simulink model "mp1"  (R2018b)
settings: Solver=VariableStepAuto  StartTime=0.0  StopTime=10.0  RelTol=1e-3
values from neighbouring files (symbols this model uses):
  b = 54.2e-6    (= 5.42e-05)    [Untitled_M65.m]
  d = 1.1e-6    (= 1.1e-06)    [Untitled_M65.m]
  g = 9.81    [Untitled_M65.m]
  I = 1.08e-6    (= 1.08e-06)    [Untitled_M65.m]
  Ix = 0.008    [Untitled_M65.m]
  Iy = 0.008    [Untitled_M65.m]
  Iz = 0.142    [Untitled_M65.m]
  L = 0.24    [Untitled_M65.m]
  m = 1    [Untitled_M65.m]
  Pos_z0 = 150    [Untitled_M65.m]
libraries: mpclib x2
settings Model: Creator=z2822  LastModifiedBy=z2822

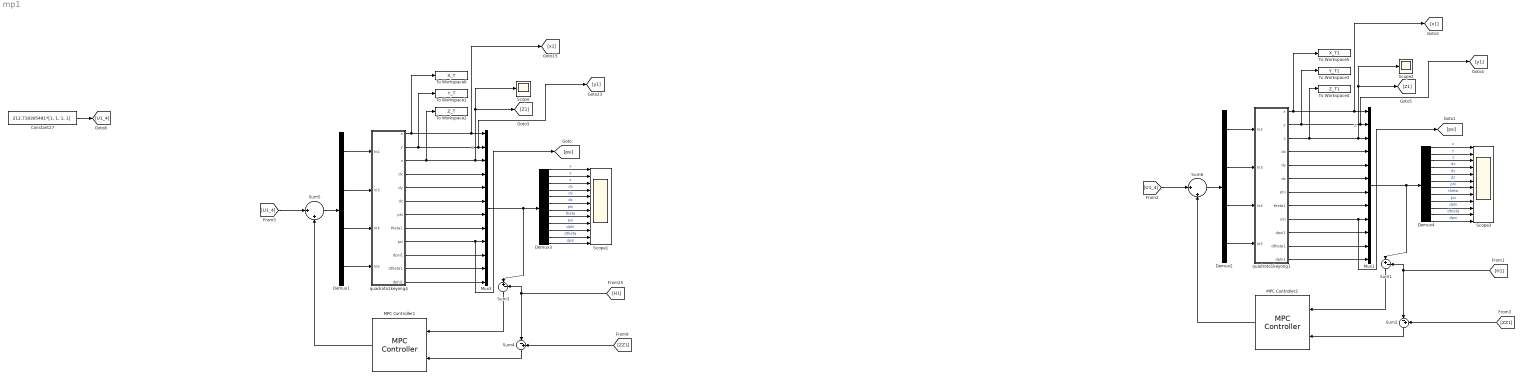
== system mp1 ==
  Constant27 : Constant  Value=212.718305491*[1, 1, 1, 1]
  Demux1 : Demux
  Demux2 : Demux
  Demux3 : Demux  Outputs=12
  Demux4 : Demux  Outputs=12
  MPC Controller1 : mpclib/MPC Controller  SCDEnableBlockLinearizationSpecification=on  mpcobj=mpc1  is_multiple=0  enable_value=0  return_u0=off  updateMPCinCallerWorkspace=on  md_inport=off  mv_inport=off  return_cost=off  return_mvseq=off  return_qpstatus=off  return_xseq=off  return_state=off  return_ovseq=off  state_inport=off  umin_inport=off  umax_inport=off  ymin_inport=off  ymax_inport=off  cc_inport=off  ywt_inport=off  uwt_inport=off  duwt_inport=off  rhoeps_inport=off  uref_inport=off  n_ts=0.83  n_p=23  n_mv=4  n_md=0  n_ud=0  n_mo=12  n_uo=0  BlockDataType=double  SampleTimeInherited=off  switch_inport=off
  MPC Controller2 : mpclib/MPC Controller  SCDEnableBlockLinearizationSpecification=on  mpcobj=mpc1  is_multiple=0  enable_value=0  return_u0=off  updateMPCinCallerWorkspace=on  md_inport=off  mv_inport=off  return_cost=off  return_mvseq=off  return_qpstatus=off  return_xseq=off  return_state=off  return_ovseq=off  state_inport=off  umin_inport=off  umax_inport=off  ymin_inport=off  ymax_inport=off  cc_inport=off  ywt_inport=off  uwt_inport=off  duwt_inport=off  rhoeps_inport=off  uref_inport=off  n_ts=0.83  n_p=23  n_mv=4  n_md=0  n_ud=0  n_mo=12  n_uo=0  BlockDataType=double  SampleTimeInherited=off  switch_inport=off
  Mux1 : Mux  Inputs=12
  Mux3 : Mux  Inputs=12
  Scope : Scope
  Scope1 : Scope  NumInputPorts=12
  Scope2 : Scope
  Scope3 : Scope  NumInputPorts=12
  Sum1 : Sum  Inputs=|+-
  Sum2 : Sum  Inputs=|-+
  Sum3 : Sum  Inputs=|+-
  Sum4 : Sum  Inputs=|-+
  Sum5 : Sum  Inputs=||+|+
  Sum6 : Sum  Inputs=||+|+
  To Workspace1 : ToWorkspace  VariableName=Y_T  SaveFormat=Timeseries  SampleTime=-1
  To Workspace2 : ToWorkspace  VariableName=Z_T  SaveFormat=Timeseries  SampleTime=-1
  To Workspace3 : ToWorkspace  VariableName=Y_T1  SaveFormat=Timeseries  SampleTime=-1
  To Workspace4 : ToWorkspace  VariableName=Z_T1  SaveFormat=Timeseries  SampleTime=-1
  To Workspace5 : ToWorkspace  VariableName=X_T1  SaveFormat=Timeseries  SampleTime=-1
  To Workspace6 : ToWorkspace  VariableName=X_T  SaveFormat=Timeseries  SampleTime=-1
  quadroto1keyong1 : Subsystem
  quadroto1keyong4 : Subsystem
  wires:
  Demux3/8 -> Scope1/8  "theta"
  Demux3/6 -> Scope1/6  "dz"
  Demux3/12 -> Scope1/12  "dpsi"
  quadroto1keyong4/12(dphi1) -> Mux3/12
  Demux3/4 -> Scope1/4  "dx"
  Demux3/9 -> Scope1/9  "psi"
  Demux3/10 -> Scope1/10  "dphi"
  Demux3/11 -> Scope1/11  "dtheta"
  quadroto1keyong4/5(dy) -> Mux3/5
  quadroto1keyong4/11(dtheta1) -> Mux3/11
  quadroto1keyong4/10(dpsi1) -> Mux3/10
  MPC Controller1/1 -> Sum5/2
  Demux3/5 -> Scope1/5  "dy"
  quadroto1keyong4/9(psi) -> [psi], Mux3/9
  Demux1/1 -> quadroto1keyong4/1(In2)
  quadroto1keyong4/2(y) -> To Workspace1/1, Mux3/2, [y1]
  [ZZ1] -> Sum4/2
  Sum4/1 -> MPC Controller1/2
  Demux1/4 -> quadroto1keyong4/4(In5)
  Demux3/1 -> Scope1/1  "x"
  Demux3/3 -> Scope1/3  "z"
  [H1] -> Sum4/1, Sum3/2
  quadroto1keyong4/7(phi) -> Mux3/7
  quadroto1keyong4/4(dx) -> Mux3/4
  Demux1/3 -> quadroto1keyong4/3(In4)
  Sum5/1 -> Demux1/1
  quadroto1keyong4/6(dz) -> Mux3/6
  quadroto1keyong4/8(theta1) -> Mux3/8
  Sum3/1 -> MPC Controller1/1
  Mux3/1 -> Sum3/1, Demux3/1
  Demux3/2 -> Scope1/2  "y"
  quadroto1keyong4/3(z) -> To Workspace2/1, Mux3/3, Scope/1, [Z1]  "Z"
  [U1_4] -> Sum5/1
  Demux3/7 -> Scope1/7  "phi"
  quadroto1keyong4/1(x) -> To Workspace6/1, Mux3/1, [x1]
  Demux1/2 -> quadroto1keyong4/2(In3)
  quadroto1keyong1/1(x) -> To Workspace5/1, Mux1/1, [x1]
  Demux4/7 -> Scope3/7  "phi"
  quadroto1keyong1/8(theta1) -> Mux1/8
  quadroto1keyong1/6(dz) -> Mux1/6
  Sum6/1 -> Demux2/1
  Demux2/3 -> quadroto1keyong1/3(In4)
  [U1_4] -> Sum6/1
  Sum1/1 -> MPC Controller2/1
  Demux4/1 -> Scope3/1  "x"
  quadroto1keyong1/3(z) -> To Workspace4/1, Mux1/3, Scope2/1, [Z1]  "Z"
  Demux4/3 -> Scope3/3  "z"
  quadroto1keyong1/4(dx) -> Mux1/4
  [ZZ1] -> Sum2/2
  Mux1/1 -> Sum1/1, Demux4/1
  quadroto1keyong1/7(phi) -> Mux1/7
  quadroto1keyong1/2(y) -> To Workspace3/1, Mux1/2, [y1]
  Demux4/9 -> Scope3/9  "psi"
  quadroto1keyong1/5(dy) -> Mux1/5
  Demux4/2 -> Scope3/2  "y"
  quadroto1keyong1/11(dtheta1) -> Mux1/11
  Demux2/1 -> quadroto1keyong1/1(In2)
  Demux4/5 -> Scope3/5  "dy"
  [H1] -> Sum2/1, Sum1/2
  Demux2/4 -> quadroto1keyong1/4(In5)
  MPC Controller2/1 -> Sum6/2
  Demux2/2 -> quadroto1keyong1/2(In3)
  quadroto1keyong1/10(dpsi1) -> Mux1/10
  Demux4/10 -> Scope3/10  "dphi"
  Demux4/11 -> Scope3/11  "dtheta"
  Demux4/6 -> Scope3/6  "dz"
  Sum2/1 -> MPC Controller2/2
  quadroto1keyong1/12(dphi1) -> Mux1/12
  quadroto1keyong1/9(psi) -> [psi], Mux1/9
  Demux4/12 -> Scope3/12  "dpsi"
  Demux4/4 -> Scope3/4  "dx"
  Demux4/8 -> Scope3/8  "theta"
  Constant27/1 -> [U1_4]

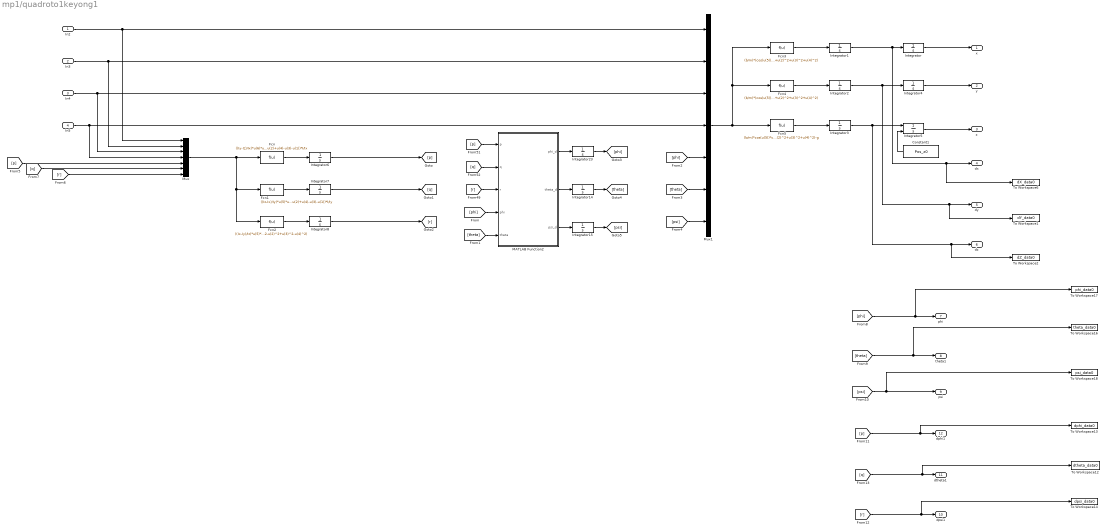
== system mp1/quadroto1keyong1 ==
  In2 : Inport
  In3 : Inport  Port=2
  In4 : Inport  Port=3
  In5 : Inport  Port=4
  Constant1 : Constant  Value=Pos_z0
  Fcn : Fcn  Expr=((Iy-Iz)/Ix)*u(6)*u(7)+(b*L/Ix)*(u(4)^2-u(2)^2)-u(6)*(u(2)+u(4)-u(3)-u(1))*I/Ix
  Fcn1 : Fcn  Expr=((Iz-Ix)/Iy)*u(5)*u(7)+(b*L/Iy)*(u(3)^2-u(1)^2)-u(5)*(u(2)+u(4)-u(3)-u(1))*I/Iy
  Fcn2 : Fcn  Expr=((Ix-Iy)/Iz)*u(5)*u(6)+(d/Iz)*(u(1)^2-u(2)^2+u(3)^2-u(4)^2)
  Fcn3 : Fcn  Expr=(b/m)*(cos(u(5))*sin(u(6))*cos(u(7))+sin(u(5))*sin(u(7)))*(u(1)^2+u(2)^2+u(3)^2+u(4)^2)
  Fcn4 : Fcn  Expr=(b/m)*(cos(u(5))*sin(u(6))*sin(u(7))-sin(u(5))*cos(u(7)))*(u(1)^2+u(2)^2+u(3)^2+u(4)^2)
  Fcn5 : Fcn  Expr=(b/m)*cos(u(5))*cos(u(6))*(u(1)^2+u(2)^2+u(3)^2+u(4)^2)-g
  Integrator{,1..4,6..8,14..15,23} (11 alike) : Integrator
  Integrator5 : Integrator  InitialConditionSource=external
  MATLAB Function2 : MATLAB Function  TreatAsAtomicUnit=on
  Mux : Mux  Inputs=7
  Mux1 : Mux  Inputs=7
  To Workspace1 : ToWorkspace  VariableName=dY_data0  SaveFormat=Timeseries  SampleTime=-1
  To Workspace12 : ToWorkspace  VariableName=dtheta_data0  SaveFormat=Timeseries  SampleTime=-1
  To Workspace13 : ToWorkspace  VariableName=dphi_data0  SaveFormat=Timeseries  SampleTime=-1
  To Workspace14 : ToWorkspace  VariableName=dpsi_data0  SaveFormat=Timeseries  SampleTime=-1
  To Workspace16 : ToWorkspace  VariableName=theta_data0  SaveFormat=Timeseries  SampleTime=-1
  To Workspace17 : ToWorkspace  VariableName=phi_data0  SaveFormat=Timeseries  SampleTime=-1
  To Workspace18 : ToWorkspace  VariableName=psi_data0  SaveFormat=Timeseries  SampleTime=-1
  To Workspace2 : ToWorkspace  VariableName=dZ_data0  SaveFormat=Timeseries  SampleTime=-1
  To Workspace6 : ToWorkspace  VariableName=dX_data0  SaveFormat=Timeseries  SampleTime=-1
  x : Outport
  y : Outport  Port=2
  z : Outport  Port=3
  dx : Outport  Port=4
  dy : Outport  Port=5
  dz : Outport  Port=6
  phi : Outport  Port=7
  theta1 : Outport  Port=8
  psi : Outport  Port=9
  dpsi1 : Outport  Port=10
  dtheta1 : Outport  Port=11
  dphi1 : Outport  Port=12
  wires:
  Integrator3/1 -> Integrator5/1, dz/1, To Workspace2/1
  Fcn4/1 -> Integrator2/1
  Integrator4/1 -> y/1
  In4/1 -> Mux1/3, Mux/3
  Integrator1/1 -> Integrator/1, To Workspace6/1, dx/1
  Mux/1 -> Fcn/1, Fcn1/1, Fcn2/1
  In3/1 -> Mux1/2, Mux/2
  Integrator5/1 -> z/1
  Mux1/1 -> Fcn3/1, Fcn4/1, Fcn5/1
  Fcn5/1 -> Integrator3/1
  Integrator2/1 -> Integrator4/1, To Workspace1/1, dy/1
  Fcn2/1 -> Integrator8/1
  In5/1 -> Mux/4, Mux1/4
  Fcn/1 -> Integrator6/1
  In2/1 -> Mux/1, Mux1/1
  Fcn1/1 -> Integrator7/1
  Integrator/1 -> x/1
  Fcn3/1 -> Integrator1/1
  Constant1/1 -> Integrator5/2
  [p] -> MATLAB Function2/1(p)
  [phi] -> Mux1/5
  Integrator23/1 -> [phi]
  [theta] -> MATLAB Function2/5(theta)
  [theta] -> Mux1/6
  MATLAB Function2/3(psi_d) -> Integrator15/1
  Integrator15/1 -> [psi]
  MATLAB Function2/2(theta_d) -> Integrator14/1
  [r] -> MATLAB Function2/3(r)
  [psi] -> Mux1/7
  [phi] -> MATLAB Function2/4(phi)
  [q] -> MATLAB Function2/2(q)
  MATLAB Function2/1(phi_d) -> Integrator23/1
  Integrator14/1 -> [theta]
  Integrator6/1 -> [p]
  Integrator7/1 -> [q]
  Integrator8/1 -> [r]
  [psi] -> psi/1, To Workspace18/1
  [phi] -> phi/1, To Workspace17/1
  [q] -> To Workspace12/1, dtheta1/1
  [r] -> To Workspace14/1, dpsi1/1
  [p] -> To Workspace13/1, dphi1/1
  [theta] -> theta1/1, To Workspace16/1
  [r] -> Mux/7
  [p] -> Mux/5
  [q] -> Mux/6

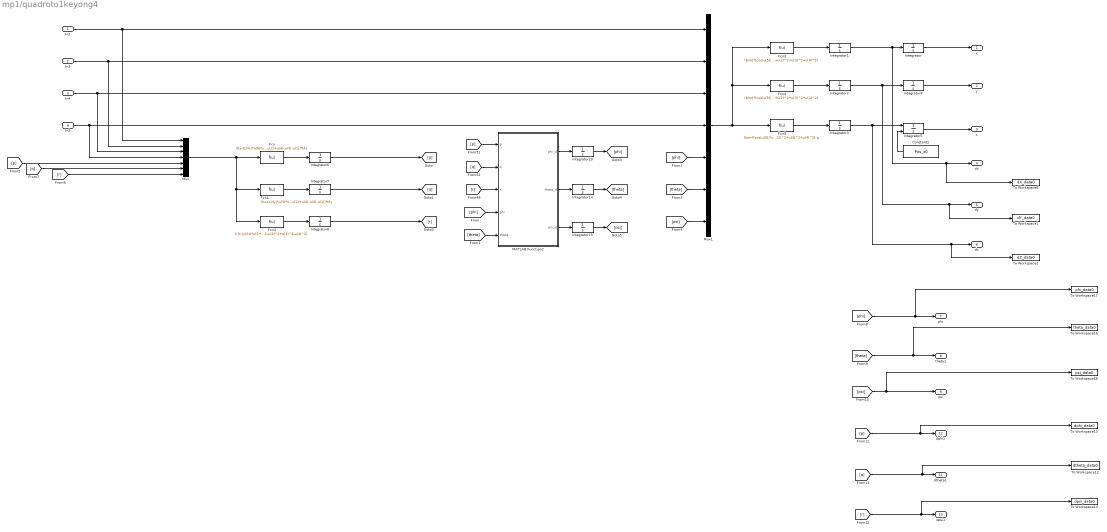
== system mp1/quadroto1keyong4 ==
  In2 : Inport
  In3 : Inport  Port=2
  In4 : Inport  Port=3
  In5 : Inport  Port=4
  Constant1 : Constant  Value=Pos_z0
  Fcn : Fcn  Expr=((Iy-Iz)/Ix)*u(6)*u(7)+(b*L/Ix)*(u(4)^2-u(2)^2)-u(6)*(u(2)+u(4)-u(3)-u(1))*I/Ix
  Fcn1 : Fcn  Expr=((Iz-Ix)/Iy)*u(5)*u(7)+(b*L/Iy)*(u(3)^2-u(1)^2)-u(5)*(u(2)+u(4)-u(3)-u(1))*I/Iy
  Fcn2 : Fcn  Expr=((Ix-Iy)/Iz)*u(5)*u(6)+(d/Iz)*(u(1)^2-u(2)^2+u(3)^2-u(4)^2)
  Fcn3 : Fcn  Expr=(b/m)*(cos(u(5))*sin(u(6))*cos(u(7))+sin(u(5))*sin(u(7)))*(u(1)^2+u(2)^2+u(3)^2+u(4)^2)
  Fcn4 : Fcn  Expr=(b/m)*(cos(u(5))*sin(u(6))*sin(u(7))-sin(u(5))*cos(u(7)))*(u(1)^2+u(2)^2+u(3)^2+u(4)^2)
  Fcn5 : Fcn  Expr=(b/m)*cos(u(5))*cos(u(6))*(u(1)^2+u(2)^2+u(3)^2+u(4)^2)-g
  Integrator{,1..4,6..8,14..15,23} (11 alike) : Integrator
  Integrator5 : Integrator  InitialConditionSource=external
  MATLAB Function2 : MATLAB Function  TreatAsAtomicUnit=on
  Mux : Mux  Inputs=7
  Mux1 : Mux  Inputs=7
  To Workspace1 : ToWorkspace  VariableName=dY_data0  SaveFormat=Timeseries  SampleTime=-1
  To Workspace12 : ToWorkspace  VariableName=dtheta_data0  SaveFormat=Timeseries  SampleTime=-1
  To Workspace13 : ToWorkspace  VariableName=dphi_data0  SaveFormat=Timeseries  SampleTime=-1
  To Workspace14 : ToWorkspace  VariableName=dpsi_data0  SaveFormat=Timeseries  SampleTime=-1
  To Workspace16 : ToWorkspace  VariableName=theta_data0  SaveFormat=Timeseries  SampleTime=-1
  To Workspace17 : ToWorkspace  VariableName=phi_data0  SaveFormat=Timeseries  SampleTime=-1
  To Workspace18 : ToWorkspace  VariableName=psi_data0  SaveFormat=Timeseries  SampleTime=-1
  To Workspace2 : ToWorkspace  VariableName=dZ_data0  SaveFormat=Timeseries  SampleTime=-1
  To Workspace6 : ToWorkspace  VariableName=dX_data0  SaveFormat=Timeseries  SampleTime=-1
  x : Outport
  y : Outport  Port=2
  z : Outport  Port=3
  dx : Outport  Port=4
  dy : Outport  Port=5
  dz : Outport  Port=6
  phi : Outport  Port=7
  theta1 : Outport  Port=8
  psi : Outport  Port=9
  dpsi1 : Outport  Port=10
  dtheta1 : Outport  Port=11
  dphi1 : Outport  Port=12
  wires:
  Integrator3/1 -> Integrator5/1, dz/1, To Workspace2/1
  Fcn4/1 -> Integrator2/1
  Integrator4/1 -> y/1
  In4/1 -> Mux1/3, Mux/3
  Integrator1/1 -> Integrator/1, To Workspace6/1, dx/1
  Mux/1 -> Fcn/1, Fcn1/1, Fcn2/1
  In3/1 -> Mux1/2, Mux/2
  Integrator5/1 -> z/1
  Mux1/1 -> Fcn3/1, Fcn4/1, Fcn5/1
  Fcn5/1 -> Integrator3/1
  Integrator2/1 -> Integrator4/1, To Workspace1/1, dy/1
  Fcn2/1 -> Integrator8/1
  In5/1 -> Mux/4, Mux1/4
  Fcn/1 -> Integrator6/1
  In2/1 -> Mux/1, Mux1/1
  Fcn1/1 -> Integrator7/1
  Integrator/1 -> x/1
  Fcn3/1 -> Integrator1/1
  Constant1/1 -> Integrator5/2
  [p] -> MATLAB Function2/1(p)
  [phi] -> Mux1/5
  Integrator23/1 -> [phi]
  [theta] -> MATLAB Function2/5(theta)
  [theta] -> Mux1/6
  MATLAB Function2/3(psi_d) -> Integrator15/1
  Integrator15/1 -> [psi]
  MATLAB Function2/2(theta_d) -> Integrator14/1
  [r] -> MATLAB Function2/3(r)
  [psi] -> Mux1/7
  [phi] -> MATLAB Function2/4(phi)
  [q] -> MATLAB Function2/2(q)
  MATLAB Function2/1(phi_d) -> Integrator23/1
  Integrator14/1 -> [theta]
  Integrator6/1 -> [p]
  Integrator7/1 -> [q]
  Integrator8/1 -> [r]
  [psi] -> psi/1, To Workspace18/1
  [phi] -> phi/1, To Workspace17/1
  [q] -> To Workspace12/1, dtheta1/1
  [r] -> To Workspace14/1, dpsi1/1
  [p] -> To Workspace13/1, dphi1/1
  [theta] -> theta1/1, To Workspace16/1
  [r] -> Mux/7
  [p] -> Mux/5
  [q] -> Mux/6

== matlab function mp1/quadroto1keyong1/MATLAB Function2 ==
  data: p input; phi_d output; q input; r input; phi input; theta input; theta_d output; psi_d output
function [phi_d, theta_d, psi_d] = fcn(p, q, r, phi, theta)


phi_d = p + q * tan(theta) * sin(phi) + r * tan(theta) * cos(phi);
theta_d = q * cos(phi) - r * sin(phi);
psi_d = (q * sin(phi) + r * cos(phi)) / cos(theta);
end

== matlab function mp1/quadroto1keyong4/MATLAB Function2 ==
  data: p input; phi_d output; q input; r input; phi input; theta input; theta_d output; psi_d output
function [phi_d, theta_d, psi_d] = fcn(p, q, r, phi, theta)


phi_d = p + q * tan(theta) * sin(phi) + r * tan(theta) * cos(phi);
theta_d = q * cos(phi) - r * sin(phi);
psi_d = (q * sin(phi) + r * cos(phi)) / cos(theta);
end
